simulink model "M05_MPC"  (R2025b)
settings: Solver=ode4  StartTime=0.01  StopTime=t_sim_stop  RelTol=1e-3
undefined symbols (not defined in the file): a, b, curvature_array, enable_obstacle, g, L, mass, max_straight_speed, mu, num_obstacles, obs_x, obs_y, path_waypoints, v_ref_array
libraries: simulink x2, autolibshared x1
settings Model: Creator=Legion  LastModifiedBy=Legion

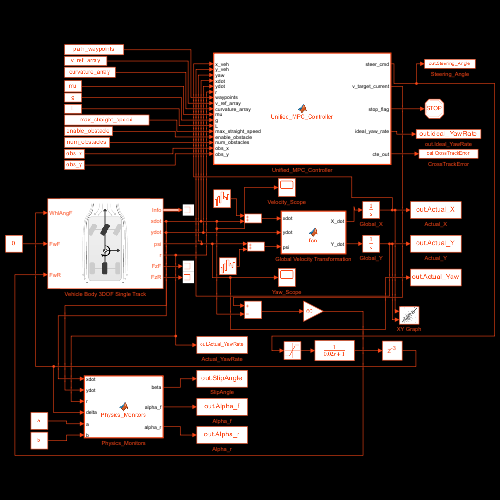
[thumbnail: Simulink's stored preview of the top-level diagram]
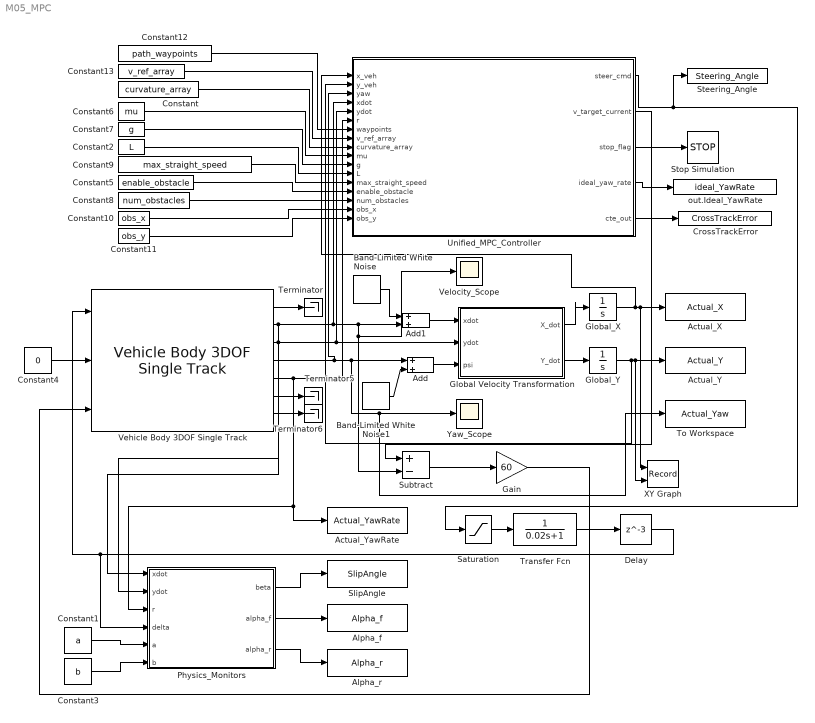
== system M05_MPC ==
  Actual_X : ToWorkspace  VariableName=Actual_X  SaveFormat=Timeseries  SampleTime=-1
  Actual_Y : ToWorkspace  VariableName=Actual_Y  SaveFormat=Timeseries  SampleTime=-1
  Actual_YawRate : ToWorkspace  VariableName=Actual_YawRate  SaveFormat=Timeseries  SampleTime=-1
  Add : Sum
  Add1 : Sum
  Alpha_f : ToWorkspace  VariableName=Alpha_f  SaveFormat=Timeseries  SampleTime=-1
  Alpha_r : ToWorkspace  VariableName=Alpha_r  SaveFormat=Timeseries  SampleTime=-1
  Band-Limited White Noise : simulink/Sources/Band-Limited White Noise  Cov=[0.0001]  Ts=0.01  seed=[23341]
  Band-Limited White Noise1 : simulink/Sources/Band-Limited White Noise  Cov=[0.0005]  Ts=0.01  seed=[23341]
  Constant : Constant  Value=curvature_array
  Constant1 : Constant  Value=a
  Constant10 : Constant  Value=obs_x
  Constant11 : Constant  Value=obs_y
  Constant12 : Constant  Value=path_waypoints
  Constant13 : Constant  Value=v_ref_array
  Constant2 : Constant  Value=L
  Constant3 : Constant  Value=b
  Constant4 : Constant  Value=0
  Constant5 : Constant  Value=enable_obstacle
  Constant6 : Constant  Value=mu
  Constant7 : Constant  Value=g
  Constant8 : Constant  Value=num_obstacles
  Constant9 : Constant  Value=max_straight_speed
  CrossTrackError : ToWorkspace  VariableName=CrossTrackError  SaveFormat=Timeseries  SampleTime=-1
  Delay : Delay  DelayLength=3
  Gain : Gain  Gain=60
  Global Velocity Transformation : MATLAB Function  TreatAsAtomicUnit=on
  Global_X : Integrator  InitialCondition=path_waypoints(1,1)
  Global_Y : Integrator  InitialCondition=path_waypoints(1,2)
  Physics_Monitors : MATLAB Function  TreatAsAtomicUnit=on
  Saturation : Saturate  UpperLimit=30 * pi/180  LowerLimit=-30 * pi/180
  SlipAngle : ToWorkspace  VariableName=SlipAngle  SaveFormat=Timeseries  SampleTime=-1
  Steering_Angle : ToWorkspace  VariableName=Steering_Angle  SaveFormat=Timeseries  SampleTime=-1
  Stop Simulation : Stop
  Subtract : Sum  Inputs=+-
  Terminator : Terminator
  Terminator5 : Terminator
  Terminator6 : Terminator
  To Workspace : ToWorkspace  VariableName=Actual_Yaw  SaveFormat=Timeseries  SampleTime=-1
  Transfer Fcn : TransferFcn  Denominator=[0.02 1]
  Unified_MPC_Controller : MATLAB Function  TreatAsAtomicUnit=on
  Vehicle Body 3DOF Single Track : autolibshared/Vehicle Body 3DOF Single Track  trackMode=Single (bicycle)  inputMode=External longitudinal forces  frontSteerMode=on  rearSteerMode=off  windMode=off  muMode=off  extFMode=off  extMMode=off  htchFMode=off  htchMMode=off  extXo=off  extpsio=off  extxdoto=off  extro=off  extYo=off  extTamb=off  extydoto=off  aMode=2  NF=2  NR=2  m=mass  a=a  b=b  h=h  dh=1  hh=0.2  X_o=0  xdot_o=0.001  CalphaMode=off  sigmaMode=off  d=0  hl=0  w=[1.4,1.4]  Cy_f=Cy_f  Cy_r=Cy_r  sigma_f=.1  sigma_r=.1  alpha_f_brk=[-0.785, -0.628, -0.471, -0.314, -0.157, 0.000, 0.157, 0.314, 0.471, 0.628, 0.785]  Cy_f_data=[2000, 3000, 4000, 5500, 7000, 9000, 7000, 5500, 4000, 3000, 2000]  alpha_r_brk=[-0.785, -0.628, -0.471, -0.314, -0.157, 0.000, 0.157, 0.314, 0.471, 0.628, 0.785]  Cy_r_data=[2000, 3000, 4000, 5500, 7000, 9000, 7000, 5500, 4000, 3000, 2000]  Y_o=0  ydot_o=0  Izz=Izz  psi_o=atan2(path_waypoints(2,2)-path_waypoints(1,2), path_waypoints(2,1)-path_waypoints(1,1))  r_o=0  Af=Af  Cd=.3  Cl=.1  Cpm=.1  beta_w=[0 0.01:0.01:0.3]  Cs=[0 0.01:0.01:0.3]  Cym=[0 1e-6:0.01:0.3]  Pabs=101325  Tair=273  g=9.81  mu=mu  xdot_tol=.01  Fznom=Fznom  Fxtire_sat=7e4  Fytire_sat=7e4  longOff=0  latOff=0  vertOff=0  wrapAng=off
  Velocity_Scope : Scope
      settings: ActiveDisplayYMinimum=0.7024131164666485  ActiveDisplayYMaximum=1.4316639746586821
  XY Graph : Record  NumPorts=2.0  FileSettingsInternal="{\"entries\":[{\"content\":{\"excelSettings\":{\"content\":{},\"type\":\"Streamout.ExcelSettings\"},\"parquetSettings\":{\"content\":{},\"type\":\"Streamout.ParquetSettings\"}},\"type\":\"Streamout.FileSettingStorage\",\"uuid\":\"\"}],\"packageUris\":[\"http:\\/\\/schema.mathworks.com\\/mf0\\/streamout_blocks\\/R2020a\"],\"version\":\"1.0\"}"  FrameSettings=[0, 0]  Layout=[1 1]  SignalsInternal="{\"entries\":[{\"content\":{\"signals\":[{\"content\":{\"blockPath\":[],\"dimensions\":[1],\"domain\":\"\",\"lineColor\":\"#fe330a\",\"lineWidth\":2,\"port\":1,\"sid\":[\"\"],\"signalID\":1,\"signalName\":\"Global_X\"},\"type\":\"RecordBlkView.Signal\",\"uuid\":\"\"},{\"content\":{\"blockPath\":[],\"dimensions\":[1],\"domain\":\"\",\"lineColor\":\"#22b573\",\"lineWidth\":2,\"port\":2,\"sid\":[\"\"],\"signalID\":2,\"signalName\":\"Global_Y\"},\"type\":\"RecordBlkView.Signal\",\"uuid\":\"\"}]},\"type\":\"RecordBlkView.InputSignals\",\"uuid\":\"\"}],\"packageUris\":[\"http:\\/\\/schema.mathworks.com\\/mf0\\/streamout_blocks\\/R2020a\"],\"version\":\"1.0\"}"  VisualizationBindings="{\"xyplotplugin\":{\"info\":[{\"series\":[],\"subplotID\":1}]}}"  CompatibilityTag=XY
  Yaw_Scope : Scope
      settings: ActiveDisplayYMinimum=-0.24426851447788056  ActiveDisplayYMaximum=1.1237341178679363
  out.Ideal_YawRate : ToWorkspace  VariableName=ideal_YawRate  SaveFormat=Timeseries  SampleTime=-1
  wires:
  Subtract/1 -> Gain/1
  Gain/1 -> Vehicle Body 3DOF Single Track/3
  Vehicle Body 3DOF Single Track/3 -> Global Velocity Transformation/2(ydot), Unified_MPC_Controller/5(ydot), Physics_Monitors/2(ydot)
  Vehicle Body 3DOF Single Track/7 -> Terminator6/1
  Saturation/1 -> Transfer Fcn/1
  Vehicle Body 3DOF Single Track/1 -> Terminator/1
  Vehicle Body 3DOF Single Track/4 -> Add/1, Yaw_Scope/1, To Workspace/1, Unified_MPC_Controller/3(yaw)
  Global Velocity Transformation/2(Y_dot) -> Global_Y/1
  Transfer Fcn/1 -> Delay/1
  Global_Y/1 -> XY Graph/2, Actual_Y/1, Unified_MPC_Controller/2(y_veh)
  Global Velocity Transformation/1(X_dot) -> Global_X/1
  Global_X/1 -> XY Graph/1, Actual_X/1, Unified_MPC_Controller/1(x_veh)
  Constant4/1 -> Vehicle Body 3DOF Single Track/2
  Vehicle Body 3DOF Single Track/6 -> Terminator5/1
  Vehicle Body 3DOF Single Track/5 -> Physics_Monitors/3(r), Actual_YawRate/1, Unified_MPC_Controller/6(r)
  Unified_MPC_Controller/1(steer_cmd) -> Saturation/1, Steering_Angle/1
  Constant2/1 -> Unified_MPC_Controller/12(L)
  Vehicle Body 3DOF Single Track/2 -> Velocity_Scope/1, Subtract/2, Add1/2, Unified_MPC_Controller/4(xdot), Physics_Monitors/1(xdot)
  Physics_Monitors/2(alpha_f) -> Alpha_f/1
  Constant1/1 -> Physics_Monitors/5(a)
  Physics_Monitors/1(beta) -> SlipAngle/1
  Physics_Monitors/3(alpha_r) -> Alpha_r/1
  Constant3/1 -> Physics_Monitors/6(b)
  Constant/1 -> Unified_MPC_Controller/9(curvature_array)
  Constant12/1 -> Unified_MPC_Controller/7(waypoints)
  Constant13/1 -> Unified_MPC_Controller/8(v_ref_array)
  Unified_MPC_Controller/3(stop_flag) -> Stop Simulation/1
  Unified_MPC_Controller/4(ideal_yaw_rate) -> out.Ideal_YawRate/1
  Add/1 -> Global Velocity Transformation/3(psi)
  Add1/1 -> Global Velocity Transformation/1(xdot)
  Band-Limited White Noise/1 -> Add1/1
  Band-Limited White Noise1/1 -> Add/2
  Delay/1 -> Physics_Monitors/4(delta), Vehicle Body 3DOF Single Track/1
  Unified_MPC_Controller/5(cte_out) -> CrossTrackError/1
  Constant6/1 -> Unified_MPC_Controller/10(mu)
  Constant7/1 -> Unified_MPC_Controller/11(g)
  Constant9/1 -> Unified_MPC_Controller/13(max_straight_speed)
  Unified_MPC_Controller/2(v_target_current) -> Subtract/1
  Constant5/1 -> Unified_MPC_Controller/14(enable_obstacle)
  Constant8/1 -> Unified_MPC_Controller/15(num_obstacles)
  Constant10/1 -> Unified_MPC_Controller/16(obs_x)
  Constant11/1 -> Unified_MPC_Controller/17(obs_y)

== matlab function M05_MPC/Physics_Monitors ==
  data: xdot input; beta output; ydot input; r input; delta input; a input; b input; alpha_f output; alpha_r output
function [beta, alpha_f, alpha_r] = Physics_Monitors(xdot, ydot, r, delta, a, b)
    % This block mathematically derives the slip angles to prove tire saturation.
    % xdot: Longitudinal velocity (m/s)
    % ydot: Lateral velocity (m/s)
    % r: Yaw rate (rad/s)
    % delta: Actual front wheel steering angle (rad)
    % a, b: Distances from CG to front/rear axles (m)

    % 1. Safety limit to prevent division by zero when starting from a standstill
    v_x_safe = max(xdot, 0.1); 

    % 2. Vehicle Slip Angle (\beta)
    % Angle between the vehicle's longitudinal axis and its actual direction of travel
    beta = atan(ydot / v_x_safe);

    % 3. Front Tire Slip Angle (\alpha_f)
    % Combines lateral velocity, yaw rotation effect (a*r), and subtracts steering angle
    alpha_f = atan((ydot + a * r) / v_x_safe) - delta;

    % 4. Rear Tire Slip Angle (\alpha_r)
    % Combines lateral velocity and yaw rotation effect (rear axle moves opposite to front during yaw)
    alpha_r = atan((ydot - b * r) / v_x_safe);
end

== matlab function M05_MPC/Global Velocity Transformation ==
  data: xdot input; X_dot output; ydot input; psi input; Y_dot output
function [X_dot, Y_dot] = fcn(xdot, ydot, psi)
    % Rotate Body Velocities into Global Map Velocities
    X_dot = xdot * cos(psi) - ydot * sin(psi);
    Y_dot = xdot * sin(psi) + ydot * cos(psi);
end

== matlab function M05_MPC/Unified_MPC_Controller ==
  settings: updateMethod=DISCRETE
  data: x_veh input; steer_cmd output; y_veh input; yaw input; xdot input; ydot input; r input; waypoints input; v_ref_array input; curvature_array input; mu input; g input; L input; max_straight_speed input; v_target_current output; stop_flag output; ideal_yaw_rate output; cte_out output; enable_obstacle input; num_obstacles input; obs_x input; obs_y input
function [steer_cmd, v_target_current, stop_flag, ideal_yaw_rate, cte_out] = Unified_MPC_Controller(x_veh, y_veh, yaw, xdot, ydot, r, waypoints, v_ref_array, curvature_array, mu, g, L, max_straight_speed, enable_obstacle, num_obstacles, obs_x, obs_y)
    % =========================================================================
    % MODEL 5: UNIFIED PREDICTIVE CONTROLLER (EXPLICIT MPC ARCHITECTURE)
    % V5.1 - Multiple Random Spatial Awareness & APF Swarm Avoidance
    % =========================================================================
    
    persistent last_idx has_finished v_target_prev r_prev ydot_prev xdot_prev;
    if isempty(last_idx), last_idx = 1; end
     if isempty(has_finished), has_finished = false; end
    if isempty(v_target_prev), v_target_prev = 0; end 
    if isempty(r_prev), r_prev = 0; end
    if isempty(ydot_prev), ydot_prev = 0; end
    if isempty(xdot_prev), xdot_prev = 0; end
    
    % Initialize outputs
    stop_flag = 0; steer_cmd = 0; v_target_current = 0; ideal_yaw_rate = 0; cte_out = 0;
    
    % 1. FINISH LINE LOGIC
    if last_idx > (length(waypoints) * 0.95)
        dx_track = waypoints(end, 1) - waypoints(end-1, 1);
        dy_track = waypoints(end, 2) - waypoints(end-1, 2);
        dx_car = x_veh - waypoints(end, 1);
        dy_car = y_veh - waypoints(end, 2); 
        if (dx_track * dx_car + dy_track * dy_car) > 0, has_finished = true; end
    end
    if has_finished, stop_flag = 1; return; end
    
    % =========================================================================
    % 2. SIGNAL FILTERING (Combating IMU & Encoder Contamination Noise)
    % =========================================================================
    lpf_alpha = 0.15; % Heavy noise rejection
    r_filt    = lpf_alpha * r    + (1 - lpf_alpha) * r_prev;
    ydot_filt = lpf_alpha * ydot + (1 - lpf_alpha) * ydot_prev;
    xdot_filt = lpf_alpha * xdot + (1 - lpf_alpha) * xdot_prev;
    
    r_prev = r_filt; ydot_prev = ydot_filt; xdot_prev = xdot_filt;
    v_safe = max(xdot_filt, 1.0);
    
    % =========================================================================
    % 3. RECEDING HORIZON LOCALIZATION (With Shortcut Bug Fix)
    % =========================================================================
    min_dist = inf; closest_idx = last_idx;
    
    % Restored FIX: Constrain the search window so the car cannot "teleport" its index
    search_window = min(size(waypoints, 1) - 1, last_idx + 50); 
    
    for i = last_idx:search_window
        d = sqrt((waypoints(i,1) - x_veh)^2 + (waypoints(i,2) - y_veh)^2);
        if d < min_dist
            min_dist = d; closest_idx = i;
        end
    end
    last_idx = closest_idx;
    
    % 4. CROSS-TRACK ERROR (CTE) & IMMEDIATE KINEMATICS
    dx = waypoints(closest_idx+1, 1) - waypoints(closest_idx, 1);
    dy = waypoints(closest_idx+1, 2) - waypoints(closest_idx, 2);
    yaw_path = atan2(dy, dx);
    immediate_kappa = curvature_array(closest_idx); 
    
    l2 = dx^2 + dy^2;
    if l2 > 0
        t = ((x_veh - waypoints(closest_idx, 1)) * dx + (y_veh - waypoints(closest_idx, 2)) * dy) / l2;
        proj_x = waypoints(closest_idx, 1) + t * dx;
        proj_y = waypoints(closest_idx, 2) + t * dy;
    else
        proj_x = waypoints(closest_idx, 1); proj_y = waypoints(closest_idx, 2);
    end
    e_mag = sqrt((x_veh - proj_x)^2 + (y_veh - proj_y)^2);
    cross_prod = dx * (y_veh - waypoints(closest_idx, 2)) - dy * (x_veh - waypoints(closest_idx, 1));
    cte_out = sign(cross_prod) * e_mag; 
    
    theta_e = yaw - yaw_path;
    theta_e = atan2(sin(theta_e), cos(theta_e)); 
    
    % =========================================================================
    % 5. LATENCY PREDICTION & HORIZON SEPARATION
    % =========================================================================
    e_dot = ydot_filt + v_safe * sin(theta_e);
    theta_e_dot = r_filt - (immediate_kappa * v_safe);
    
    t_delay = 0.03; % 30ms latency cancellation
    cte_pred = cte_out + (e_dot * t_delay);
    theta_e_pred = theta_e + (theta_e_dot * t_delay);
    
    % VELOCITY PREVIEW HORIZON 
    lookahead_time = 0.65; % DECREASED: Drive deeper into straights before braking!
    lookahead_dist = v_safe * lookahead_time;
    idx_offset = round(lookahead_dist / 0.05); 
    target_idx = min(size(waypoints, 1), closest_idx + idx_offset);
    target_kappa = curvature_array(target_idx); 
    
    ideal_yaw_rate = immediate_kappa * v_safe;
    
    % 6. KAMM FRICTION CIRCLE (Velocity Target)
    if abs(target_kappa) > 1e-4
        v_friction_limit = sqrt((mu * g) / abs(target_kappa));
    else
        v_friction_limit = max_straight_speed;
    end
    v_target_base = min([v_ref_array(target_idx), v_friction_limit, max_straight_speed]);
    
    % =========================================================================
    % 7. PREDICTIVE STEERING LAW (Robust LPV Scheduling)
    % =========================================================================
    k_e     = 1.0 + (8.0 / v_safe);     
    k_theta = 1.5 + (10.0 / v_safe); 
    k_edot  = 0.2 + (2.0 / v_safe); 
    k_rdot  = 0.1 + (1.0 / v_safe);  
    
    steer_ff = atan(immediate_kappa * L);
    steer_fb = - (k_e * cte_pred) - (k_theta * theta_e_pred) - (k_edot * e_dot) - (k_rdot * theta_e_dot);
    
    % =========================================================================
    % 8. MULTI-OBSTACLE ARTIFICIAL POTENTIAL FIELD (APF)
    % =========================================================================
    steer_repulsion = 0;
    
    if enable_obstacle == 1
        influence_radius = 8.0; % Start dodging 8 meters away
        
        for k = 1:num_obstacles
            d_obs = sqrt((x_veh - obs_x(k))^2 + (y_veh - obs_y(k))^2);
            
            if d_obs < influence_radius
                % Calculate angle to obstacle relative to car's current heading
                yaw_obs = atan2(obs_y(k) - y_veh, obs_x(k) - x_veh);
                angle_diff = yaw_obs - yaw;
                angle_diff = atan2(sin(angle_diff), cos(angle_diff)); % Wrap to [-pi, pi]
                
                % React only to obstacles immediately in front (+/- 90 deg)
                if abs(angle_diff) < (pi/2)
                    % Bias dead-center approaches to force a safer right-hand pass
                    if abs(angle_diff) < 0.05
                        angle_diff = 0.05;
                    end
                    
                    % Accumulate Inverse-square repulsive forces from all nearby obstacles
                    repulsion_gain = 3.5;
                    steer_repulsion = steer_repulsion - sign(angle_diff) * (repulsion_gain / max(d_obs, 1.0)^2);
                    
                    % Dynamic Braking: Automatically slow down for the evasive maneuver!
                    v_target_base = min(v_target_base, 4.5);
                end
            end
        end
    end
    
    raw_steer_cmd = steer_ff + steer_fb + steer_repulsion;
    
    % Mechanical Actuator Limits (+/- 30 degrees)
    max_steer_rad = 30 * (pi / 180);
    steer_cmd = max(-max_steer_rad, min(max_steer_rad, raw_steer_cmd));
    
    % =========================================================================
    % 9. ELECTRONIC STABILITY CONTROL (Asymmetric & Deadband)
    % =========================================================================
    max_alpha_rad = 5 * (pi / 180);
    a_dist = 0.617 * L; 
    predicted_slip = steer_cmd - (ydot_filt + a_dist*r_filt) / v_safe;
    
    % FEATURE 1: The Steering Deadband
    steer_deadband = 2 * (pi / 180); 
    
    if abs(steer_cmd) > steer_deadband && abs(predicted_slip) > max_alpha_rad
        v_req = v_target_base * 0.70; 
    else
        v_req = v_target_base; 
    end
    
    % FEATURE 2: Asymmetric Alpha Smoothing (RACING LINE CALIBRATION)
    if v_req < v_target_prev
        alpha_filter = 0.85; % BRAKE FAST: 85% immediate weight transfer
    else
        alpha_filter = 0.10; % ACCELERATE 5X FASTER: Eat up the short straights!
    end
    
    v_target_current = (alpha_filter * v_req) + ((1 - alpha_filter) * v_target_prev);
    v_target_prev = v_target_current;
end
